simulink model "single_reservoir"  (R2020b)
settings: Solver=VariableStepAuto  StartTime=0.0  StopTime=t  RelTol=1e-3
values from neighbouring files (symbols this model uses):
  A1 = 1    [init_single_reservoir.m]
  Aout = 0.1    [init_single_reservoir.m]
  g = 9.81    [init_single_reservoir.m]
  H1 = 10    [init_single_reservoir.m]
settings Model: Creator=root  LastModifiedBy=root

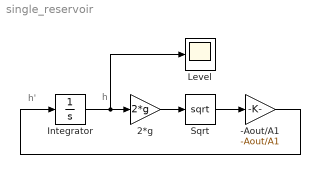
== system single_reservoir ==
  note: h'
  note: h
  -Aout/A1 : Gain  Gain=-Aout/A1
  2*g : Gain  Gain=2*g
  Integrator : Integrator  InitialCondition=H1
  Level : Scope
  Sqrt : Sqrt  SaturateOnIntegerOverflow=on
  wires:
  -Aout/A1/1 -> Integrator/1
  2*g/1 -> Sqrt/1
  Integrator/1 -> 2*g/1, Level/1
  Sqrt/1 -> -Aout/A1/1
